simulink model "TrayectoriaEvitaObstaculos"  (R2023b)
settings: Solver=FixedStepAuto  StartTime=0.0  StopTime=150  RelTol=1e-3  EnableMultiTasking=on
model workspace (MAT data in the model file):
  d = 0.21
libraries: robotalgslib x1
settings Model: ExtModeTrigDuration=2  Creator=Felix  LastModifiedBy=Daniel
settings OptimizationCC: EnhancedBackFolding=on  PassReuseOutputArgsAs=Individual arguments  ZeroExternalMemoryAtStartup=off  ZeroInternalMemoryAtStartup=off  MaxStackSize=64  OptimizeBlockOrder=speed  DifferentSizesBufferReuse=on  EfficientTunableParamExpr=on
settings DebuggingCC: ParameterTunabilityLossMsg=error
settings HardwareCC: ProdBitPerInt=16  ProdBitPerPointer=16  ProdBitPerSizeT=16  ProdBitPerPtrDiffT=16  ProdLargestAtomicFloat=None  ProdWordSize=8  ProdHWDeviceType=Atmel->AVR
settings SFSimCC: MATLABDynamicMemAlloc=off
settings RTWCC: Description=Embedded Coder  SystemTargetFile=ert.tlc  HardwareBoard=Arduino Mega 2560  TemplateMakefile=ert_default_tmf  Toolchain=Arduino AVR  BuildConfiguration=Faster Runs
settings CodeAppCC: ForceParamTrailComments=on  IgnoreCustomStorageClasses=off  OperatorAnnotations=on  SimulinkDataObjDesc=on  SFDataObjDesc=on  InsertBlockDesc=on
settings ERTTargetCC: SupportContinuousTime=on  SupportVariableSizeSignals=on  ExtModeTransport=3  ExtModeStaticAlloc=on  ExtModeAutomaticAllocSize=off  ExtModeStaticAllocSize=2048  ExtModeMexFile=ext_xcp  ExtModeIntrfLevel=Level2 - Open

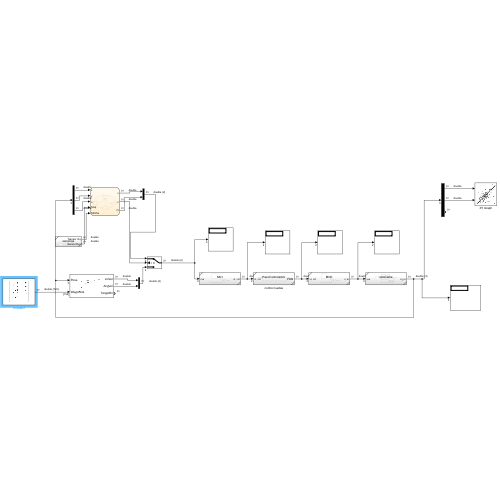
[thumbnail: Simulink's stored preview of the top-level diagram]
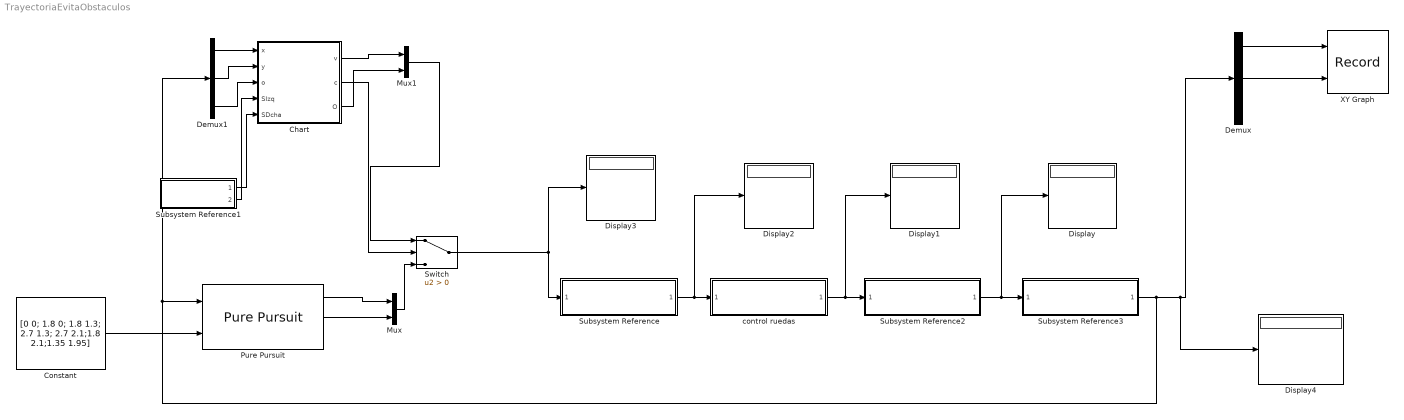
== system TrayectoriaEvitaObstaculos ==
  Chart : Stateflow chart  TreatAsAtomicUnit=on
  Constant : Constant  Value=[0 0; 1.8 0; 1.8 1.3; 2.7 1.3; 2.7 2.1;1.8 2.1;1.35 1.95]
  Demux : Demux  Outputs=3
  Demux1 : Demux  Outputs=3
  Display{,1..4} (5 alike) : Display
  Mux : Mux  Inputs=2
  Mux1 : Mux  Inputs=2
  Pure Pursuit : robotalgslib/Pure Pursuit  DesiredLinearVelocity=0.18  MaxAngularVelocity=0.75  LookaheadDistance=0.3  TargetDirPort=on  SimulateUsing=Code generation
      settings: LibrarySourceBlock=robotmobilelib/Pure Pursuit
  Subsystem Reference : Subsystem  ReferencedSubsystem=MCI
  Subsystem Reference1 : Subsystem  ReferencedSubsystem=sensores
  Subsystem Reference2 : Subsystem  ReferencedSubsystem=MCD
  Subsystem Reference3 : Subsystem  ReferencedSubsystem=odometria
  Switch : Switch  Criteria=u2 > Threshold  SaturateOnIntegerOverflow=off  InputSameDT=off
  XY Graph : Record  FileSettingsInternal="{\"entries\":[{\"content\":{\"excelSettings\":{\"content\":{},\"type\":\"Streamout.ExcelSettings\"}},\"type\":\"Streamout.FileSettingStorage\",\"uuid\":\"\"}],\"packageUris\":[\"http:\\/\\/schema.mathworks.com\\/mf0\\/streamout_blocks\\/R2020a\"],\"version\":\"1.0\"}"  Layout=[1 1]  SignalsInternal="{\"entries\":[{\"content\":{\"signals\":[{\"content\":{\"blockPath\":[],\"dimensions\":[1],\"domain\":\"\",\"lineColor\":\"#a2142f\",\"plots\":[ 1 ],\"port\":1,\"signalID\":1,\"signalName\":\"Demux:1\"},\"type\":\"RecordBlkView.Signal\",\"uuid\":\"\"},{\"content\":{\"blockPath\":[],\"dimensions\":[1],\"domain\":\"\",\"lineColor\":\"#139fff\",\"plots\":[ 1 ],\"port\":2,\"signalID\":2,\"signalName\":\"Demux:2\"},\"type\":\"RecordBlkView.Signal\",\"uuid\":\"\"}]},\"type\":\"RecordBlkView.InputSignals\",\"uuid\":\"\"}],\"packageUris\":[\"http:\\/\\/schema.mathworks.com\\/mf0\\/streamout_blocks\\/R2020a\"],\"version\":\"1.0\"}"  VisualizationBindings="{\"xyplotplugin\":{\"info\":[{\"series\":[{\"bindingParametersList\":[{\"parameter\":\"X-Axis\",\"signalID\":1,\"signalName\":\"Demux:1\"},{\"parameter\":\"Y-Axis\",\"signalID\":2,\"signalName\":\"Demux:2\"}],\"seriesID\":0}],\"subplotID\":1}]}}"  CompatibilityTag=XY
  control ruedas : Subsystem  ReferencedSubsystem=PieroControladoV
  wires:
  Switch/1 -> Subsystem Reference/1, Display3/1
  Subsystem Reference/1 -> Display2/1, control ruedas/1
  control ruedas/1 -> Display1/1, Subsystem Reference2/1
  Subsystem Reference2/1 -> Display/1, Subsystem Reference3/1
  Subsystem Reference3/1 -> Pure Pursuit/1, Demux1/1, Demux/1, Display4/1
  Demux/1 -> XY Graph/1
  Demux/2 -> XY Graph/2
  Pure Pursuit/1 -> Mux/1
  Constant/1 -> Pure Pursuit/2
  Pure Pursuit/2 -> Mux/2
  Mux/1 -> Switch/3
  Demux1/1 -> Chart/1(x)
  Demux1/2 -> Chart/2(y)
  Demux1/3 -> Chart/3(o)
  Chart/2(c) -> Switch/2
  Chart/1(v) -> Mux1/1
  Mux1/1 -> Switch/1
  Subsystem Reference1/1 -> Chart/5(SDcha)
  Subsystem Reference1/2 -> Chart/4(SIzq)
  Chart/3(O) -> Mux1/2

== stateflow chart TrayectoriaEvitaObstaculos/Chart ==
  state SinObstaculo
    v=0;
    O=0;
    c=0;
  state ObstaculoDer
    v=0.1;
    O=pi/4;
    c=1;
  state ObstaculoIzq
    v=0.1;
    O=-pi/4;
    c=1;
  state ObstaculoFrente
    v=0;
    O=pi/2;
    c=1;
  (default) -> SinObstaculo
  SinObstaculo -> ObstaculoIzq [order 2] : [SDcha<20]
  SinObstaculo -> ObstaculoDer [order 1] : [SIzq<20]
  ObstaculoDer -> SinObstaculo [order 1] : after(1,sec)
  ObstaculoFrente -> SinObstaculo : after(2,sec)
  ObstaculoIzq -> SinObstaculo [order 1] : after(1,sec)
  ObstaculoDer -> ObstaculoFrente [order 2] : [SDcha<15]
  ObstaculoIzq -> ObstaculoFrente [order 2] : [SIzq<15]
  data: v output double size=1; c output size=1; O output size=1; x input size=1; y input size=1; o input size=1; SIzq input size=1; SDcha input size=1
